simulink model "SimulinkStartExample"  (R2026a)
settings: Solver=VariableStepAuto  StopTime=10
settings Model: Creator=UmarMuslimBinMohdFay  LastModifiedBy=UmarMuslimBinMohdFay

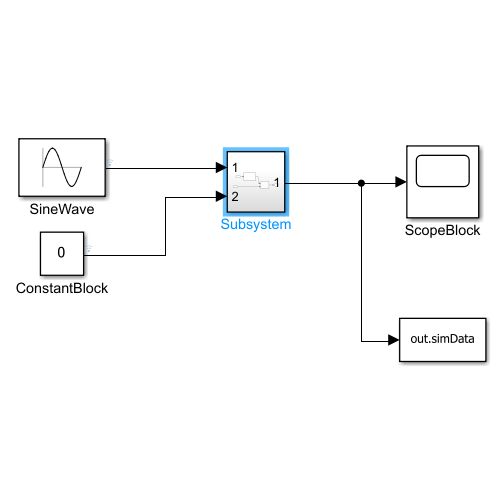
[thumbnail: Simulink's stored preview of the top-level diagram]
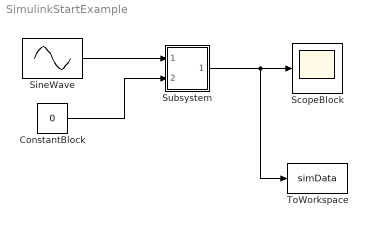
== system SimulinkStartExample ==
  ConstantBlock : Constant  Value=0
  ScopeBlock : Scope
      settings: ActiveDisplayYMinimum=-4.2393778240309512  ActiveDisplayYMaximum=3.2473984350306782
  SineWave : Sin  Frequency=2  SampleTime=0
  Subsystem : Subsystem
  ToWorkspace : ToWorkspace  VariableName=simData  SaveFormat=Structure With Time  SampleTime=-1
  wires:
  Subsystem/1(Out1) -> ToWorkspace/1, ScopeBlock/1
  SineWave/1 -> Subsystem/1(In1)
  ConstantBlock/1 -> Subsystem/2(In2)

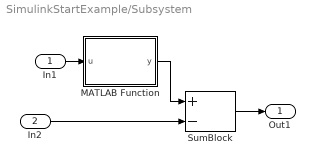
== system SimulinkStartExample/Subsystem ==
  In1 : Inport
  In2 : Inport  Port=2
  MATLAB Function : MATLAB Function  TreatAsAtomicUnit=on
  SumBlock : Sum  Inputs=+-
  Out1 : Outport
  wires:
  SumBlock/1 -> Out1/1
  In2/1 -> SumBlock/2
  In1/1 -> MATLAB Function/1(u)
  MATLAB Function/1(y) -> SumBlock/1

== matlab function SimulinkStartExample/Subsystem/MATLAB Function ==
  data: u input; y output
function y = fcn(u)
    y = 2*u;
